simulink model "test_emplanner_cs"  (R2021a)
settings: Solver=ode5  StartTime=0.0  StopTime=120  FixedStep=1/1000  RelTol=1e-3
PreLoadFcn:
  | mbxruntime.callbacks.PreLoadFcn(bdroot);
PostLoadFcn:
  | mbxruntime.callbacks.PostLoadFcn(bdroot);
InitFcn:
  | mbxruntime.callbacks.InitFcn(bdroot);
StartFcn:
  | mbxruntime.callbacks.StartFcn(bdroot);
StopFcn:
  | mbxruntime.callbacks.StopFcn(bdroot);
model workspace (MAT data in the model file):
  mbox_table : object (value not decoded)
  model_closed = 0
  sim_status = 0
values from neighbouring files (symbols this model uses):
  c_factor = 43.75    [emplanner_init.m]
  cf = -175016    [emplanner_init.m]
  cr = -130634    [emplanner_init.m]
  global_path_x = [-2.7494 -1.75001774493 -0.751894634419 0.244952249347 1.24051712279 2.23479835808 3.22779585569 4.21951007764 5.20994169183 6.19909144113 7.18696009523 8.17354843293 ... (3001 elements, 3001x1)]    [global_path.mat]
  global_path_y = [18.2589 18.2589 18.2589 18.2589 18.2589 18.2589 18.2589 18.2589 18.2589 18.2589 18.2589 18.2589 ... (3001 elements, 3001x1)]    [global_path.mat]
  KD_PID_distance = 0.0    (= 0)    [emplanner_init.m]
  KD_PID_speed = 0    [emplanner_init.m]
  KI_PID_distance = 0.0    (= 0)    [emplanner_init.m]
  KI_PID_speed = 0    [emplanner_init.m]
  KP_PID_distance = 0.5    [emplanner_init.m]
  KP_PID_speed = 1.8    [emplanner_init.m]
  la = 1.265    [emplanner_init.m]
  lb = 2.947-1.265    (= 1.682)    [emplanner_init.m]
  LQR_K1 = k(:,1)'    [emplanner_init.m]
  LQR_K2 = k(:,2)'    [emplanner_init.m]
  LQR_K3 = k(:,3)'    [emplanner_init.m]
  LQR_K4 = k(:,4)'    [emplanner_init.m]
  m = 2020    [emplanner_init.m]
  rack_displacement = [-39.14 , -37.2 , -35.29 , -33.43 , -31.6 , -29.81 , -28.06 , -26.34 , -24.66 ,      -23.01 , -21.38 , -19.79 , -18.23 , -16.69 , -15.18 , -13.7 , -12.23 , -10.8 , -9.38 , -7.98 ,     -6.61 , -5.25 , -3.91 , -2.59 , -1.29 , 0 , 1.27 , 2.54 , 3.78 , 5.02 , 6.24 , 7.46 , 8.66 ,      9.86 , 11.05 , 12.24 , 13.41 , 14.59 , 15.76 , 16.92 , 18.09 , 19.25 , 20.42 , 21.59 , 22.76 ,      23.93 , 25.11 , 26 ...(+26 chars)    [emplanner_init.m]
  right_wheel_ground = [-70 ,-67.2 , -64.4 , -61.6 , -58.8 , -56 , -53.2 , -50.4 , -47.6 , -44.8 , -42 ,      -39.2 , -36.4 , -33.6 , -30.8 , -28 , -25.2 , -22.4 , -19.6 , -16.8 , -14 , -11.2 , -8.4 , -5.6 ,      -2.8 , 0 , 2.8 , 5.6 , 8.4 , 11.2 , 14 , 16.8 , 19.6 , 22.4 , 25.2 , 28 , 30.8 , 33.6 , 36.4 ,      39.2 , 42 , 44.8 , 47.6 , 50.4 , 53.2 , 56 , 58.8 , 61.6 , 64.4 , 67.2 , 70 ]    [emplanner_init.m]
  vx_break_point = zeros(1,5000)    [emplanner_init.m]
undefined symbols (not defined in the file or in its folder): aubr, DiscIntNeverNeededParam, tablebr, vubr, warningInitialVelocity, x0
libraries: PreScanSimulinkLibrary x27, simulink x19, simulink_extras x6, Solver_SF x1
(part 11 of 11)

== matlab function test_emplanner_cs/Audi_A8_Sedan_1/decision&planning module/referenceline provider/mine_tou ==
  data: x_set input; match_point_index_set output; y_set input; frenet_path_x_set input; frenet_path_y_set input; frenet_path_heading_set input; proj_x_set output; proj_y_set output; proj_heading_set output; proj_kappa_set output; frenet_path_kappa_set input
function [match_point_index_set,proj_x_set,proj_y_set,proj_heading_set,proj_kappa_set] =...
    fcn(x_set,y_set,frenet_path_x_set,frenet_path_y_set,frenet_path_heading_set,frenet_path_kappa_set)
%不知道输出集合个数，预设为128个
n=128;
match_point_index_set=ones(n,1)*nan;
proj_x_set=ones(n,1)*nan;
proj_y_set=ones(n,1)*nan;
proj_heading_set=ones(n,1)*nan;
proj_kappa_set=ones(n,1)*nan;
%申明全局变量
persistent is_first_run;
persistent pre_match_point_index_set;
persistent pre_frenet_path_x_set;
persistent pre_frenet_path_y_set;
persistent pre_frenet_path_heading_set;
persistent pre_frenet_path_kappa_set;
persistent pre_x_set;
persistent pre_y_set;
if isempty(is_first_run)
    %首次运行
    is_first_run=0;
    pre_frenet_path_x_set = frenet_path_x_set;
    pre_frenet_path_y_set = frenet_path_y_set;
    pre_frenet_path_heading_set = frenet_path_heading_set;
    pre_frenet_path_kappa_set = frenet_path_kappa_set;
    pre_match_point_index_set=ones(n,1)*nan;
    for i=1:length(x_set)
        if isnan(x_set(i))
            break;
        end
        %首次运行，从第一个点开始找
        start_search_index=1;
        %用于记录distance连续增加个数
        increase_count=0;
        min_distance=inf;%假设最小距离为无穷大
        for j=start_search_index:length(frenet_path_x_set)
            distance=(x_set(i)-frenet_path_x_set(j))^2+(y_set(i)-frenet_path_y_set(j))^2;
            if distance<min_distance
                min_distance=distance;
                match_point_index_set(i)=j;
                increase_count=0;
            else
                increase_count=increase_count+1;
            end
            if increase_count>50
                 break;
            end
        end
        %通过匹配点计算投影点
        %取出匹配点编号
        match_point_index=match_point_index_set(i);
        %取出匹配点信息
        match_point_x=frenet_path_x_set(match_point_index);
        match_point_y=frenet_path_y_set(match_point_index);
        match_point_heading=frenet_path_heading_set(match_point_index);
        match_point_kappa=frenet_path_kappa_set(match_point_index);
        %计算匹配点的位置向量和方向向量
        vector_match_point=[match_point_x;match_point_y];
        vector_match_point_direction=[cos(match_point_heading);sin(match_point_heading)];
        %待投影点的位置向量
        vector_r=[x_set(i);y_set(i)];
        %通过匹配点计算
        vector_d=vector_r-vector_match_point;
        ds=vector_d'*vector_match_point_direction;
        vector_proj_point=vector_match_point+ds*vector_match_point_direction;
        proj_heading=match_point_heading+match_point_kappa*ds;
        proj_kappa=match_point_kappa;

        %合并输出结果
        proj_x_set(i)=vector_proj_point(1);
        proj_y_set(i)=vector_proj_point(2);
        proj_heading_set(i)=proj_heading;
        proj_kappa_set(i)=proj_kappa;
     end
     %匹配点计算结果保存，供下一个计算周期使用
     pre_match_point_index_set=match_point_index_set;
     pre_x_set=x_set;
     pre_y_set=y_set;
else
    %非首次运行
    for i=1:length(x_set)
        start_search_index=pre_match_point_index_set(i);
        %判断帧与帧之间的障碍物是否为同一个
        square_dis=(x_set(i)-pre_x_set(i))^2+(y_set(i)-pre_y_set(i))^2;
        if square_dis>36
            start_search_index=nan;
        end
        %对于障碍物检测而言，当感知第一次检测到障碍物时，算法不是首次运行，此时pre_match_point_index_set的值为nan，
        %如果还用上一时刻的结果作为本周期搜索起点，会出问题，进行修改
        %声明increase_count_limit
        increase_count_limit=5;
        if isnan(start_search_index)
            %没有上个周期的结果，不能只检查5次
            increase_count_limit=50;
            %搜索起点设为1
            start_search_index=1;
        end
        %用于记录distance连续增加个数
        increase_count=0;
        %判断遍历方向
        %计算上个周期的匹配点位失，前提条件是frenet的道路信息不变，参考线模块是不变的，其他模块的参考线平滑是不断变化的，因此不能作为通用模块
        vector_pre_match_point=[frenet_path_x_set(start_search_index);frenet_path_y_set(start_search_index)];
        vector_pre_match_point_direction=...
            [cos(frenet_path_heading_set(start_search_index));sin(frenet_path_heading_set(start_search_index))];
        flag=([x_set(i);y_set(i)]-vector_pre_match_point)'*vector_pre_match_point_direction;
        min_distance=inf;%假设最小距离为无穷大
        if flag>0.001
             for j=start_search_index:length(frenet_path_x_set)
                 distance=(x_set(i)-frenet_path_x_set(j))^2+(y_set(i)-frenet_path_y_set(j))^2;
                 if distance<min_distance
                    min_distance=distance;
                    match_point_index_set(i)=j;
                    increase_count=0;
                 else
                    increase_count=increase_count+1;
                 end
                 if increase_count>increase_count_limit
                     break;
                 end
             end
        elseif flag<-0.001
            for j=start_search_index:-1:1
              distance=(x_set(i)-frenet_path_x_set(j))^2+(y_set(i)-frenet_path_y_set(j))^2;
              if distance<min_distance
                  min_distance=distance;
                  match_point_index_set(i)=j;
                  increase_count=0;
              else
                  increase_count=increase_count+1;
               end
                if increase_count>increase_count_limit
                    break;
                end
            end
        else
            match_point_index_set(i) = start_search_index;
        end
        %通过匹配点计算投影点
        %取出匹配点编号
        match_point_index=match_point_index_set(i);
        %取出匹配点信息
        match_point_x=frenet_path_x_set(match_point_index);
        match_point_y=frenet_path_y_set(match_point_index);
        match_point_heading=frenet_path_heading_set(match_point_index);
        match_point_kappa=frenet_path_kappa_set(match_point_index);
        %计算匹配点的位置向量和方向向量
        vector_match_point=[match_point_x;match_point_y];
        vector_match_point_direction=[cos(match_point_heading);sin(match_point_heading)];
        %待投影点的位置向量
        vector_r=[x_set(i);y_set(i)];
        %通过匹配点计算
        vector_d=vector_r-vector_match_point;
        ds=vector_d'*vector_match_point_direction;
        vector_proj_point=vector_match_point+ds*vector_match_point_direction;
        proj_heading=match_point_heading+match_point_kappa*ds;
        proj_kappa=match_point_kappa;
        %合并输出结果
        proj_x_set(i)=vector_proj_point(1);
        proj_y_set(i)=vector_proj_point(2);
        proj_heading_set(i)=proj_heading;
        proj_kappa_set(i)=proj_kappa;
    end
    %匹配点计算结果保存，供下一个计算周期使用
    pre_match_point_index_set=match_point_index_set;
    pre_frenet_path_x_set = frenet_path_x_set;
    pre_frenet_path_y_set = frenet_path_y_set;
    pre_frenet_path_heading_set = frenet_path_heading_set;
    pre_frenet_path_kappa_set = frenet_path_kappa_set;
    pre_x_set=x_set;
    pre_y_set=y_set;
end
end
